simulink model "regulator_LQR_discrete_COMPARISON"  (R2023a)
settings: Solver=VariableStepAuto  StartTime=0.0  StopTime=0.06  RelTol=1e-3
values from neighbouring files (symbols this model uses):
  B_tilda = [sysdis.B(1) Bw_bar(1,1) Bw_bar(1,2); sysdis.B(2) Bw_bar(2,1) Bw_bar(2,2)]    [motor.m]
  D_tilda = [0 0 0 ; 0 0 0]    [motor.m]
  sysdis = c2d(sys,Ts)    [motor.m]
  Ts = 0.001    [parameters.m]
  u_max = 12    [constraints.m]
  u_min = 0    [constraints.m]
  uBar = -(A(1,1)*(-A(2,2)*nref/A(2,1)) + A(1,2)*nref)*L    [motor.m]
  x0 = [0.2 70.3]'    [motor.m]
  yref = [iref nref]'    [motor.m]
undefined symbols (not defined in the file or in its folder): Kd, Kd1, Kd2, Kd3
settings Model: Creator=teora  LastModifiedBy=Diego

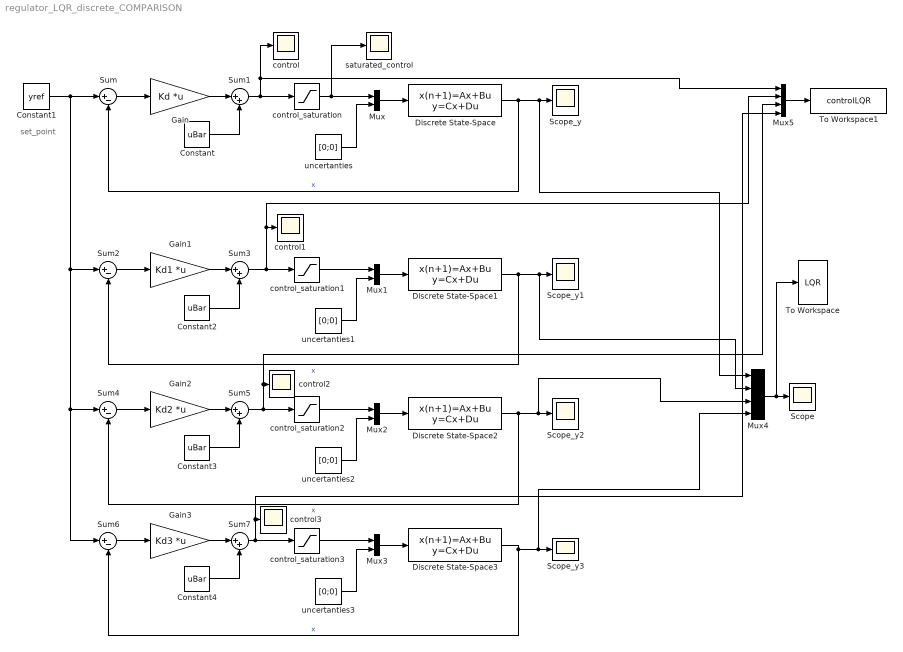
== system regulator_LQR_discrete_COMPARISON ==
  note: set_point
  Constant{,2..4} (4 alike) : Constant  Value=uBar
  Constant1 : Constant  Value=yref
  Discrete State-Space{,1..3} (4 alike) : DiscreteStateSpace  A=sysdis.A  B=B_tilda  C=sysdis.C  D=D_tilda  InitialCondition=x0  SampleTime=Ts
  Gain : Gain  Gain=Kd  Multiplication=Matrix(K*u)
  Gain1 : Gain  Gain=Kd1  Multiplication=Matrix(K*u)
  Gain2 : Gain  Gain=Kd2  Multiplication=Matrix(K*u)
  Gain3 : Gain  Gain=Kd3  Multiplication=Matrix(K*u)
  Mux{,1..3} (4 alike) : Mux  Inputs=2
  Mux4 : Mux
  Mux5 : Mux
  Scope : Scope
  Scope_y{,1..3} (4 alike) : Scope
  Sum{,2,4,6} (4 alike) : Sum  Inputs=|+-
  Sum{1,3,5,7} (4 alike) : Sum  Inputs=|++
  To Workspace : ToWorkspace  VariableName=LQR  SaveFormat=Timeseries  SampleTime=-1
  To Workspace1 : ToWorkspace  VariableName=controlLQR  SaveFormat=Timeseries  SampleTime=-1
  control{,1..3} (4 alike) : Scope
  control_saturation{,1..3} (4 alike) : Saturate  UpperLimit=u_max  LowerLimit=u_min
  saturated_control : Scope
  uncertanties{,1..3} (4 alike) : Constant  Value=[0;0]
  wires:
  Mux5/1 -> To Workspace1/1
  control_saturation3/1 -> Mux3/1
  Discrete State-Space3/1 -> Mux4/4, Scope_y3/1, Sum6/2  "x"
  Mux3/1 -> Discrete State-Space3/1
  Constant4/1 -> Sum7/2
  uncertanties3/1 -> Mux3/2
  Constant3/1 -> Sum5/2
  Sum5/1 -> Mux5/3, control2/1, control_saturation2/1
  uncertanties2/1 -> Mux2/2
  control_saturation2/1 -> Mux2/1
  Mux4/1 -> To Workspace/1, Scope/1
  uncertanties1/1 -> Mux1/2
  Sum4/1 -> Gain2/1
  Mux1/1 -> Discrete State-Space1/1
  control_saturation1/1 -> Mux1/1
  Discrete State-Space1/1 -> Mux4/2, Scope_y1/1, Sum2/2  "x"
  Sum3/1 -> Mux5/2, control1/1, control_saturation1/1
  Gain1/1 -> Sum3/1
  Gain2/1 -> Sum5/1
  Mux2/1 -> Discrete State-Space2/1
  Sum2/1 -> Gain1/1
  Discrete State-Space2/1 -> Mux4/3, Scope_y2/1, Sum4/2  "x"
  Constant2/1 -> Sum3/2
  Gain3/1 -> Sum7/1
  Constant/1 -> Sum1/2
  Sum1/1 -> Mux5/1, control/1, control_saturation/1
  Mux/1 -> Discrete State-Space/1
  Discrete State-Space/1 -> Mux4/1, Scope_y/1, Sum/2  "x"
  Sum7/1 -> Mux5/4, control3/1, control_saturation3/1
  Gain/1 -> Sum1/1
  Constant1/1 -> Sum6/1, Sum4/1, Sum2/1, Sum/1
  Sum6/1 -> Gain3/1
  Sum/1 -> Gain/1
  control_saturation/1 -> Mux/1, saturated_control/1
  uncertanties/1 -> Mux/2
